simulink model "six_01"  (R2021a)
settings: Solver=FixedStepDiscrete  StartTime=0.0  StopTime=300  FixedStep=0.1  RelTol=1e-3  EnableMultiTasking=on
settings Model: Creator=AlgoOy  LastModifiedBy=AlgoOy
settings SolverCC: AlgebraicLoopSolver=TrustRegion  AutoInsertRateTranBlk=on
settings DataIOCC: LimitDataPoints=on
settings OptimizationCC: LifeSpan=inf
settings DebuggingCC: AllowSymbolicDim=off  SFUnexpectedBacktrackingDiag=warning  SFNoUnconditionalDefaultTransitionDiag=warning  SFExecutionAtInitializationDiag=none  ArithmeticOperatorsInVariantConditions=warning
settings SFSimCC: SimUseLocalCustomCode=off  CustomCodeUndefinedFunction=UseInterfaceOnly
settings RTWCC: RTWUseLocalCustomCode=off
settings CodeAppCC: StateflowObjectComments=on
settings GRTTargetCC: TargetLangStandard=C89/C90 (ANSI)
settings ConfigComp: CovMetricSettings=dw  CovSaveCumulativeToWorkspaceVar=on  CovSaveSingleToWorkspaceVar=on  CovExternalEMLEnable=off

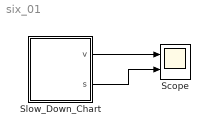
== system six_01 ==
  Scope : Scope  NumInputPorts=2
  Slow_Down_Chart : Stateflow chart  TreatAsAtomicUnit=on
  wires:
  Slow_Down_Chart/1(v) -> Scope/1
  Slow_Down_Chart/2(s) -> Scope/2

== stateflow chart six_01/Slow_Down_Chart ==
  state UD
    entry:
    t = 0;
    v = v0;
    s = s0;
    during:
    t = t + 0.01;
    v = v0 - 1.35 * t;
    s = s + 0.01 * v;
  state SD
    entry:
    t = 0;
    during:
    t = t + 0.01;
    v = 0.045 * t * t - 4.36 * t + v0;
    s = s + 0.01 * v;
  state STOP
    entry:
    v = 0;
  (default) -> UD : {s0 = 0;
      | v0 = 27.78;}
  UD -> SD : [v <= 5.56]{v0 = v}
  SD -> STOP : [v <= 0]
  data: v output; s output; t local; v0 local; s0 local
